simulink model "GEMM_Ex1"  (R2025a)
settings: Solver=VariableStepAuto  StartTime=0.0  StopTime=10  RelTol=1e-3
undefined symbols (not defined in the file): Correlation_ValidMode, DUT, L, major, Row, vsva1596, xcvc1702
libraries: aieDSP x1, aieUtilities x1, vmcUtilities x1
settings Model: Creator=sdegala  LastModifiedBy=sdegala
settings ModelReferenceCC: EnableRefExpFcnMdlSchedulingChecks=on
settings RTWCC: GPUComputeCapability=3.5

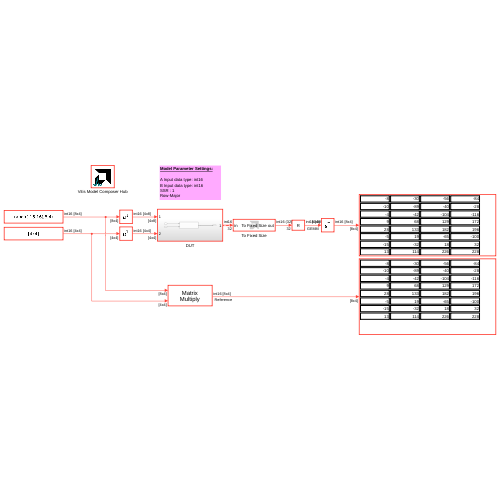
[thumbnail: Simulink's stored preview of the top-level diagram]
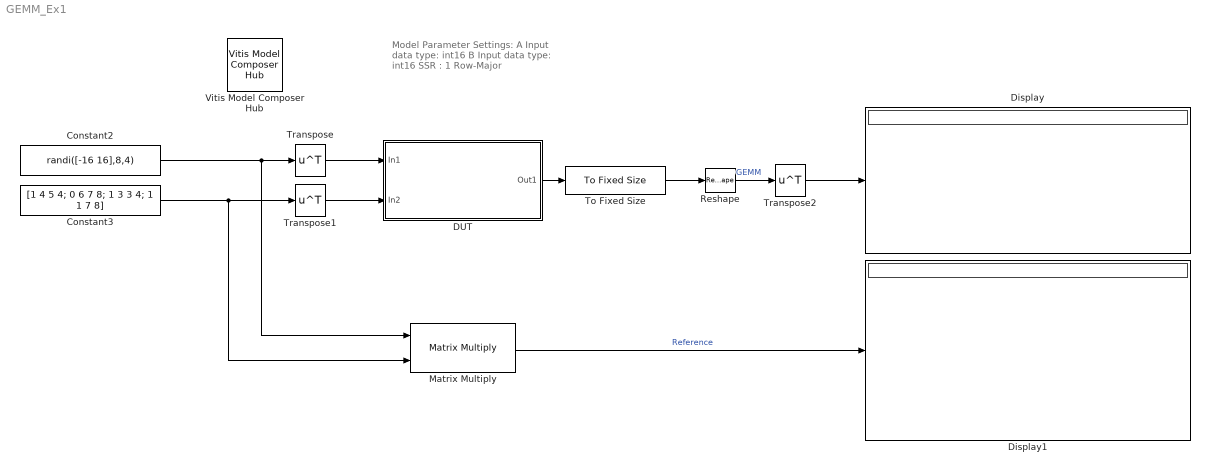
== system GEMM_Ex1 ==
  note: Model Parameter Settings:
      |
      | A Input data type: int16
      | B Input data type: int16
      | SSR : 1
      | Row-Major
  Constant2 : Constant  Value=randi([-16 16],8,4)  OutDataTypeStr=int16  SampleTime=1
  Constant3 : Constant  Value=[1 4 5 4; 0 6 7 8; 1 3 3 4; 1 1 7 8]  OutDataTypeStr=int16  SampleTime=1
  DUT : Subsystem
  Display : Display
  Display1 : Display
  Matrix Multiply : Product  Multiplication=Matrix(*)  OutDataTypeStr=int16
  Reshape : Reshape  OutputDimensionality=Customize  OutputDimensions=[4,8]
  To Fixed Size : aieUtilities/To Fixed Size  Mode=Stop simulation when input variable-size signal is not full  OutputSize=Inherit: Same as input  CopyMethod=Buffer samples to form output  HasStatusOutput=on
  Transpose : Math  Operator=transpose
  Transpose1 : Math  Operator=transpose
  Transpose2 : Math  Operator=transpose
  Vitis Model Composer Hub : vmcUtilities/Vitis Model Composer Hub  Tag=genX  CodeGeneration=off  SubsystemName=DUT  BlockHierPath=Correlation_ValidMode/DUT  SubsystemType=AIENode  StartColumn=1  NumberOfColumns=1  TargetDirectory=./code  exportDesign=off  analyzeDesign=on  validateDesignOnHw=off  ExportType=AI Engines  IpVendor=xilinx.com  IpLibrary=hls  IpVersion=1.0  IpHWLanguage=Verilog  AieCompilerOptions={}  AieSimulatorOptions={}  CreateTestbench=on  TestbenchStackSize=10  RunRtlSim=off  RunCSim=off  RunAieSim=off  AieSimTimeout=50000  RunAieSimProfiling=off  LaunchVitisAnalyzer=off  PlotOutput=off  RunX86Sim=off  X86SimTimeout=10  GenHwImage=off  GenLibadfXo=off  GenHwValidationCode=off  PlatformType=Not Specified  HwSystemType=Baremetal  HwValidationTarget=hw  ProjDevice=xcvc1702-vsva1596-2LP-e-L  ProjDevicePart=xcvc1702-vsva1596-2LP-e-L  AIEType=AIE  SamplePeriod=-1  ClockFrequency=200  DataPathParallelism=1  xilinxfamily=versalaicore  part=xcvc1702  speed=-2LP-e-L  package=vsva1596  directory=./netlist  testbench=off  incr_netlist=off  synthesis_tool=Vivado  clock_wrapper=Clock Enables  dbl_ovrd=According to Block Masks  dcm_input_clock_period=10  sysclk_period=10  simulink_period=1  eval_field=0  IPInfoJsonString="{\"DUTSubsystemName\":\"DUT\",\"AIESubsystem\":{\"SubsystemName\":\"DUT\",\"TargetDirectory\":\"./code\",\"AIEArrayConfig\":\"Use entire AIE array\",\"StartColumn\":\"0\",\"NumberOfColumns\":\"1\"},\"SubsystemTag\":\"AIENode\"}"  LogFileName=/proj/xhdhdstaff5/sdegala/Head1/HEAD/2025_2_work/AIE_BLOCKS_2025_2/code/model_composer.log  NThreads=4  IPConfigFile=/tmp/vmctmp-11198269997411262707/Correlation_ValidMode_ipconfig.json
  wires:
  Constant3/1 -> Transpose1/1, Matrix Multiply/2
  Constant2/1 -> Transpose/1, Matrix Multiply/1
  Matrix Multiply/1 -> Display1/1  "Reference"
  DUT/1(Out1) -> To Fixed Size/1
  Reshape/1 -> Transpose2/1  "GEMM"
  To Fixed Size/1 -> Reshape/1
  Transpose/1 -> DUT/1(In1)
  Transpose1/1 -> DUT/2(In2)
  Transpose2/1 -> Display/1

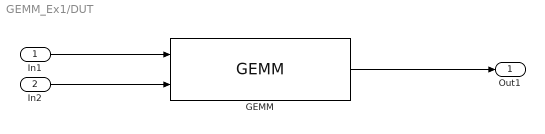
== system GEMM_Ex1/DUT ==
  In1 : Inport
  In2 : Inport  Port=2
  GEMM : aieDSP/GEMM  AIE_VARIANT=1  data_type_A=int16  data_type_B=int16  data_type_out=int16  Dim_A=8  Dim_B=4  Dim_AB=4  ssr=1  casc_length=1  InputWindowSizeA=32  InputWindowSizeB=16  A_Leading_data=Row-major(0)  B_Leading_data=Row-major(0)  Output_Leading_data=Row-major(0)  A_Tiling_data=off  B_Tiling_data=off  Output_Detiling_data=off  shift_output=0  rnd_mode=Floor  sat_mode=None  blockJsonConstraints=[]  blockJsonConstraintsInternal=[]  spec=vmc_matrix_mult.json  SerializedMaskParamNames=[]  SerializedMaskParamValues=[]  SerializedMaskParamVisibilities=[]  block_type=GEMM  SerializedMaskParamDataypes=uint|typename|typename|typename|uint|uint|uint|uint|uint|uint|uint|uint|uint|uint|uint|uint|uint|uint|uint|uint  SerializedMaskParamEnumStrArr=0|0|0|0|0|0|0|0|0|0|0|Row-major(0),Column-major(1)|Row-major(0),Column-major(1)|Row-major(0),Column-major(1)|0|0|0|0|Floor,Ceiling,Round to positive infinity,Round to negative infinity,Round symmetrical to infinity,Round symmetrical to zero,Round convergent to even,Round convergent to odd|None,Saturate,Symmetric  SerializedMaskParamEnumValArr=0|0|0|0|0|0|0|0|0|0|0|0,1|0,1|0,1|0|0|0|0|0,1,2,3,4,5,6,7|0,1,3  SerializedMaskParamVectorArr=0|0|0|0|0|0|0|0|0|0|0|0|0|0|0|0|0|0|0|0  SerializedMaskParamKeys=AIE_VARIANT|TT_DATA_A|TT_DATA_B|TT_OUT_DATA|TP_DIM_A|TP_DIM_B|TP_DIM_AB|TP_SSR|TP_CASC_LEN|TP_INPUT_WINDOW_VSIZE_A|TP_INPUT_WINDOW_VSIZE_B|TP_DIM_A_LEADING|TP_DIM_B_LEADING|TP_DIM_OUT_LEADING|TP_ADD_TILING_A|TP_ADD_TILING_B|TP_ADD_DETILING_OUT|TP_SHIFT|TP_RND|TP_SAT
  Out1 : Outport
  wires:
  In2/1 -> GEMM/2
  In1/1 -> GEMM/1
  GEMM/1 -> Out1/1
